simulink model "V90_2MW_TurbineModel_26_11_2021"  (R2020a)
settings: Solver=VariableStepAuto  StartTime=0.0  StopTime=10  RelTol=1e-3  EnableMultiTasking=on
model workspace (MAT data in the model file):
  Tw : Simulink.Parameter (value not decoded)
  c : Simulink.Parameter (value not decoded)
  dcm : Simulink.Parameter (value not decoded)
  r : Simulink.Parameter (value not decoded)
values from neighbouring files (symbols this model uses):
  N = 100    [Generator_specs.m]
  s = tf('s')    [Wind_Turbine_Pitch.m]
symbols that are objects in the model workspace (value not decoded): c, dcm, r, Tw
undefined symbols (not defined in the file or in its folder): T, X, Y, Z
libraries: sm_lib x21, nesl_utility x12, fl_lib x5, aerolibtransform2 x3, aerolibwind2 x3, aerolib6dof2 x1, simulink x1, aerolibasang x1
(part 2 of 2)

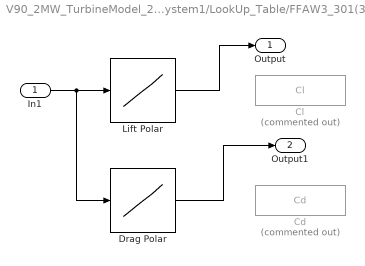
== system V90_2MW_TurbineModel_26_11_2021/Subsystem1/LookUp_Table/FFAW3_301(3to8) ==
  In1 : Inport
  Cd : ToWorkspace  Commented=on  VariableName=Cd  SampleTime=-1
      settings: Save2DSignal=2-D array (concatenate along first dimension)
  Cl : ToWorkspace  Commented=on  VariableName=Cl  SampleTime=-1
      settings: Save2DSignal=2-D array (concatenate along first dimension)
  Drag Polar : Lookup_n-D  NumberOfTableDimensions=1  BreakpointsForDimension1=|  Table=|  InternalRulePriority=Speed  RndMeth=Simplest  InputSameDT=on
      BreakpointsForDimension1=|
      | [0.095846645
      | 0.623003195
      | 1.150159744
      | 1.629392971
      | 2.156549521
      | 2.68370607
      | 3.21086262
      | 3.785942492
      | 4.217252396
      | 4.600638978
      | 5.079872204
      | 5.702875399
      | 6.42172524
      | 7.284345048
      | 7.955271565
      | 8.722044728
      | 9.440894569
      | 10.25559105
      | 10.97444089
      | 11.59744409
      | 12.22044728
      | 12.65175719
      | 13.22683706
      | 13.84984026
      | 14.47284345
      | 15.14376997
      | 15.67092652
      | 16.24600639
      | 16.77316294
      | 17.20447284
      | 17.73162939
      | 18.25878594
      | 18.78594249
      | 19.60063898
      | 20.51118211
      | 21.27795527
      | 21.85303514
      | 22.57188498
      | 23.09904153
      | 23.67412141
      | 24.34504792
      | 24.82428115
      | 25.44728435
      | 25.87859425
      | 26.45367412
      | 26.8370607
      | 27.50798722]
      Table=|
      | [0.050561798
      | 0.049297753
      | 0.049297753
      | 0.049297753
      | 0.049297753
      | 0.048033708
      | 0.049297753
      | 0.049297753
      | 0.050561798
      | 0.050561798
      | 0.050561798
      | 0.050561798
      | 0.051825843
      | 0.051825843
      | 0.053089888
      | 0.054353933
      | 0.061938202
      | 0.074578652
      | 0.079634831
      | 0.092275281
      | 0.094803371
      | 0.097331461
      | 0.10238764
      | 0.1125
      | 0.118820225
      | 0.131460674
      | 0.136516854
      | 0.149157303
      | 0.160533708
      | 0.168117978
      | 0.173174157
      | 0.180758427
      | 0.188342697
      | 0.198455056
      | 0.208567416
      | 0.211095506
      | 0.213623596
      | 0.218679775
      | 0.223735955
      | 0.228792135
      | 0.23258427
      | 0.238904494
      | 0.243960674
      | 0.247752809
      | 0.249016854
      | 0.252808989
      | 0.256601124]
  Lift Polar : Lookup_n-D  NumberOfTableDimensions=1  BreakpointsForDimension1=|  Table=|  InternalRulePriority=Speed  RndMeth=Simplest  InputSameDT=on
      BreakpointsForDimension1=|
      | [0.142857143
      | 0.571428571
      | 1.047619048
      | 1.428571429
      | 1.80952381
      | 2.238095238
      | 2.571428571
      | 2.904761905
      | 3.238095238
      | 3.666666667
      | 4.095238095
      | 4.333333333
      | 4.714285714
      | 5.142857143
      | 5.428571429
      | 5.904761905
      | 6.380952381
      | 6.80952381
      | 7.285714286
      | 7.714285714
      | 8.238095238
      | 8.761904762
      | 9.238095238
      | 10.04761905
      | 10.66666667
      | 11.23809524
      | 11.80952381
      | 12.23809524
      | 12.85714286
      | 13.23809524
      | 13.95238095
      | 14.61904762
      | 15.19047619
      | 15.71428571
      | 16.52380952
      | 17.04761905
      | 17.71428571
      | 18.28571429
      | 18.80952381
      | 19.38095238
      | 19.9047619
      | 20.57142857
      | 21.04761905
      | 21.66666667
      | 22.0952381
      | 22.57142857
      | 23.04761905
      | 23.80952381
      | 24.33333333
      | 25.14285714
      | 25.9047619
      | 26.33333333
      | 26.95238095
      | 27.33333333
      | 27.71428571]
      Table=|
      | [0.175722543
      | 0.249710983
      | 0.295953757
      | 0.351445087
      | 0.411560694
      | 0.467052023
      | 0.499421965
      | 0.54566474
      | 0.587283237
      | 0.638150289
      | 0.684393064
      | 0.726011561
      | 0.767630058
      | 0.804624277
      | 0.860115607
      | 0.897109827
      | 0.952601156
      | 0.989595376
      | 1.031213873
      | 1.07283237
      | 1.114450867
      | 1.146820809
      | 1.165317919
      | 1.165317919
      | 1.151445087
      | 1.156069364
      | 1.183815029
      | 1.211560694
      | 1.230057803
      | 1.267052023
      | 1.280924855
      | 1.299421965
      | 1.304046243
      | 1.313294798
      | 1.304046243
      | 1.29017341
      | 1.271676301
      | 1.253179191
      | 1.225433526
      | 1.202312139
      | 1.179190751
      | 1.165317919
      | 1.165317919
      | 1.156069364
      | 1.132947977
      | 1.132947977
      | 1.119075145
      | 1.058959538
      | 1.049710983
      | 1.01734104
      | 0.989595376
      | 0.975722543
      | 0.952601156
      | 0.929479769
      | 0.906358382]
  Output : Outport
  Output1 : Outport  Port=2
  wires:
  In1/1 -> Drag Polar/1, Lift Polar/1
  Drag Polar/1 -> Output1/1
  Lift Polar/1 -> Output/1

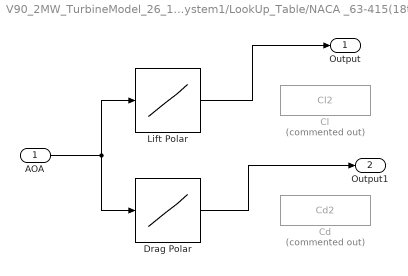
== system V90_2MW_TurbineModel_26_11_2021/Subsystem1/LookUp_Table/NACA _63-415(18to25) ==
  AOA : Inport
  Cd : ToWorkspace  Commented=on  VariableName=Cd2  SampleTime=-1
      settings: Save2DSignal=2-D array (concatenate along first dimension)
  Cl : ToWorkspace  Commented=on  VariableName=Cl2  SampleTime=-1
      settings: Save2DSignal=2-D array (concatenate along first dimension)
  Drag Polar : Lookup_n-D  NumberOfTableDimensions=1  BreakpointsForDimension1=|  Table=|  InternalRulePriority=Speed  RndMeth=Simplest  InputSameDT=on
      BreakpointsForDimension1=|
      | [0.032626427
      | 0.619902121
      | 1.305057096
      | 1.76182708
      | 2.251223491
      | 2.740619902
      | 3.099510604
      | 3.654159869
      | 4.208809135
      | 4.730831974
      | 5.187601958
      | 5.709624796
      | 6.427406199
      | 6.982055465
      | 7.569331158
      | 8.156606852
      | 8.646003263
      | 9.037520392
      | 9.657422512
      | 9.983686786
      | 10.57096248
      | 10.99510604
      | 11.45187602
      | 11.87601958
      | 12.30016313
      | 12.62642741
      | 13.01794454
      | 13.37683524]
      Table=|
      | [0.004635762
      | 0.005099338
      | 0.004635762
      | 0.004635762
      | 0.005099338
      | 0.004635762
      | 0.005562914
      | 0.005562914
      | 0.005562914
      | 0.007417219
      | 0.008344371
      | 0.008344371
      | 0.009735099
      | 0.011125828
      | 0.011125828
      | 0.01205298
      | 0.013907285
      | 0.014834437
      | 0.015298013
      | 0.014834437
      | 0.016225166
      | 0.020860927
      | 0.023178808
      | 0.026887417
      | 0.031523179
      | 0.037086093
      | 0.03986755
      | 0.047284768]
  Lift Polar : Lookup_n-D  NumberOfTableDimensions=1  BreakpointsForDimension1=|  Table=|  InternalRulePriority=Speed  RndMeth=Simplest  InputSameDT=on
      BreakpointsForDimension1=|
      | [0.093603744
      | 0.468018721
      | 0.904836193
      | 1.341653666
      | 1.684867395
      | 2.152886115
      | 2.55850234
      | 3.088923557
      | 3.556942278
      | 4.149765991
      | 4.586583463
      | 4.898595944
      | 5.335413417
      | 5.772230889
      | 6.115444618
      | 6.458658346
      | 6.833073323
      | 7.238689548
      | 7.613104524
      | 7.925117005
      | 8.361934477
      | 8.767550702
      | 9.110764431
      | 9.516380655
      | 9.953198128
      | 10.35881435
      | 10.76443058
      | 11.07644306
      | 11.45085803
      | 12.0124805
      | 12.51170047
      | 12.94851794
      | 13.32293292
      | 13.75975039
      | 14.25897036
      | 14.60218409
      | 14.97659906
      | 15.38221529
      | 15.75663027
      | 16.00624025
      | 16.16224649]
      Table=|
      | [0.369230769
      | 0.432692308
      | 0.473076923
      | 0.530769231
      | 0.576923077
      | 0.623076923
      | 0.657692308
      | 0.709615385
      | 0.773076923
      | 0.807692308
      | 0.876923077
      | 0.923076923
      | 0.963461538
      | 0.992307692
      | 1.009615385
      | 1.05
      | 1.090384615
      | 1.125
      | 1.165384615
      | 1.2
      | 1.246153846
      | 1.280769231
      | 1.309615385
      | 1.35
      | 1.373076923
      | 1.407692308
      | 1.436538462
      | 1.465384615
      | 1.476923077
      | 1.5
      | 1.528846154
      | 1.546153846
      | 1.557692308
      | 1.546153846
      | 1.546153846
      | 1.523076923
      | 1.5
      | 1.482692308
      | 1.476923077
      | 1.459615385
      | 1.442307692]
  Output : Outport
  Output1 : Outport  Port=2
  wires:
  Lift Polar/1 -> Output/1
  Drag Polar/1 -> Output1/1
  AOA/1 -> Lift Polar/1, Drag Polar/1

== matlab function V90_2MW_TurbineModel_26_11_2021/Subsystem1/Lift//Drag/MATLAB Function ==
  data: c output; Vr input; ci input; Cl input; Cl2 input; Cl3 input; dL output; FA input
function [c,dL]  = fcn(Vr,ci,Cl, Cl2, Cl3,FA)
% dL  = B*0.5*rho*Vr^2*ci*Cl
B   = 3;                                  %No. of Blades
rho = 1.2;                                %density of air in kg/m3
k   = B*0.5*rho;
c=zeros(25,1);
for i= 1:length(Cl)
    if i>=3 && i<9
        c(i,1)=Cl(i,1);
    elseif i>=9 && i<18
        c(i,1)=Cl2(i,1);
    elseif i>=18
        c(i,1)=Cl3(i,1);
    end
    %fprintf('i=%f c=%f',i,c)
dL  = k.*Vr.*Vr.*ci.*c.*sin(FA) ; 
end

== matlab function V90_2MW_TurbineModel_26_11_2021/Subsystem1/Lift//Drag/MATLAB Function1 ==
  data: D output; Vr input; ci input; Cd input; Cd2 input; Cd3 input; dD output; FA input
function [D,dD]   = fcn(Vr,ci,Cd,Cd2,Cd3,FA)
% dD  = B*0.5*rho*Vr^2*ci*Cd
B   = 3;                                  %No. of Blades
rho = 1.2;                                %density of air in kg/m3
k   = B*0.5*rho;
D=zeros(25,1);
for i= 1:length(Cd)
    if i>=3 && i<9
        D(i,1)=Cd(i,1);
    elseif i>=9 && i<18
        D(i,1)=Cd2(i,1);
    elseif i>=18
        D(i,1)=Cd3(i,1);
    end
    %fprintf('i=%f c=%f',i,c)
dD  = k.*Vr.*Vr.*ci.*D.*cos(FA); 
end

== matlab function V90_2MW_TurbineModel_26_11_2021/Subsystem1/Torque/Total Torque ==
  data: r input; dQ input; Torq output
function Torq = fcn(r, dQ)

Torq = trapz(r,dQ);
end

== matlab function V90_2MW_TurbineModel_26_11_2021/Subsystem1/Wind angle/MATLAB Function ==
  data: a output; r input; ch input; c input; D input; FAc input; ad output
function [a,ad]  = fcn(r,ch,c,D,FAc)
B = 3;                          % No. of Blades
R = 45;                         % Rotor Radius
s = (B.*ch)./(2.*pi.*r);
Cn = (c.*cos(FAc))+(D.*sin(FAc));
Ct = (c.*sin(FAc))-(D.*cos(FAc));
F  = (2/pi)*acos((exp(-((B/2).*(1-(r./R)))./((r./R).*sin(FAc)))));
%z  = exp(-((B/2).*(1-(r./R)))./((r./R).*sin(FAc));
% Axial Induction Factor

a = 1./((4.*F.*sin(FAc).*sin(FAc))./(s.*Cn)+1);
a(1) = 0.21952;
a(2) = 0.21952;
a(25) = a(24);

% Tangential Induction Factor

ad = 1./((4.*F.*sin(FAc).*cos(FAc))./(s.*Ct)-1);
ad(1) = 0.17397;
ad(2) = 0.17397;
ad(25) = ad(24);

end

== matlab function V90_2MW_TurbineModel_26_11_2021/Subsystem1/Flapwise_BM/MATLAB Function ==
  data: V input; BM_Flap output; x input
function BM_Flap = fcn(V,x)         % x= radial distance of Blade

rho = 1.2                            %Air density  in kg/m3
L   = x(length(x));                  %Blade Length

BM_Flap  = (4*rho*V*V*pi.*((2*L)+x).*(L-x).*(L-x))./81   %*(L-x)*(L-x))/81;
end

== matlab function V90_2MW_TurbineModel_26_11_2021/Subsystem1/Edgewise_BM/MATLAB Function ==
  data: x input; Edge_BM output
function Edge_BM = fcn(x)           % x= radial distance


g  = 9.81;              % in m/s2
L  = x(length(x));
m_per_blade = 5388;     % in Kg(taken from reference)

Edge_BM = m_per_blade*g*L/2
end

== matlab function V90_2MW_TurbineModel_26_11_2021/Subsystem1/Wind_Model/DCM_WT ==
  data: ya input; a14 output; tilt input; ba input; cone input
function a14 = fcn(ya,tilt,ba,cone)

a1  =[1 0 0;0 cos(ya) sin(ya);0 -sin(ya) cos(ya)];
a2  =[cos(tilt) 0 -sin(tilt);0 1 0;sin(tilt) 0 cos(tilt)];
a3  =[1 0 0;0 1 0;0 0 1];

a12 = a3*a2*a1;

a23 =[cos(ba) sin(ba) 0;-sin(ba) cos(ba) 0;0 0 1];

a34 =[cos(cone) 0 -sin(cone);0 1 0;sin(cone) 0 cos(cone)];

a14 = a34*a23*a12;
end
